simulink model "Ejemplo52"  (R2021a)
settings: Solver=ode4  StartTime=0.0  StopTime=20  FixedStep=0.01  RelTol=1e-3
settings Model: PauseTimes=10  Creator=benja  LastModifiedBy=benja

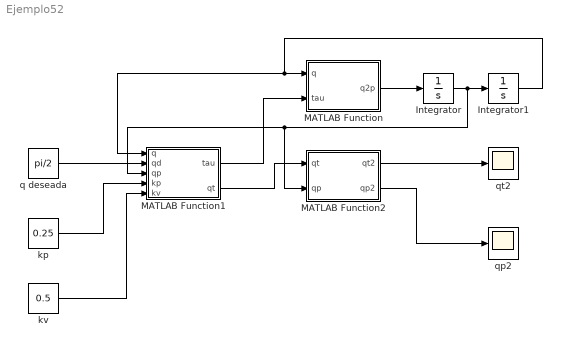
== system Ejemplo52 ==
  Integrator : Integrator
  Integrator1 : Integrator
  MATLAB Function : MATLAB Function  TreatAsAtomicUnit=on
  MATLAB Function1 : MATLAB Function  TreatAsAtomicUnit=on
  MATLAB Function2 : MATLAB Function  TreatAsAtomicUnit=on
  kp : Constant  Value=0.25
  kv : Constant  Value=0.5
  q deseada : Constant  Value=pi/2
  qp2 : Scope
  qt2 : Scope
  wires:
  MATLAB Function/1(q2p) -> Integrator/1
  Integrator/1 -> MATLAB Function2/2(qp), MATLAB Function1/3(qp), Integrator1/1
  Integrator1/1 -> MATLAB Function1/1(q), MATLAB Function/1(q)
  MATLAB Function1/1(tau) -> MATLAB Function/2(tau)
  q deseada/1 -> MATLAB Function1/2(qd)
  kp/1 -> MATLAB Function1/4(kp)
  kv/1 -> MATLAB Function1/5(kv)
  MATLAB Function2/2(qp2) -> qp2/1
  MATLAB Function1/2(qt) -> MATLAB Function2/1(qt)
  MATLAB Function2/1(qt2) -> qt2/1

== matlab function Ejemplo52/MATLAB Function1 ==
  data: q input; tau output; qd input; qp input; kp input; kv input; qt output
function [tau,qt] = fcn(q,qd,qp,kp,kv)

qt = qd - q;
tau = kp*qt-kv*qp;

== matlab function Ejemplo52/MATLAB Function ==
  data: q input; q2p output; tau input
function q2p = fcn(q,tau)

m = 1;
g = 1;
l = 1;
q2p =inv(m*l)*(tau-m*g*l*sin(q));

== matlab function Ejemplo52/MATLAB Function2 ==
  data: qt input; qt2 output; qp input; qp2 output
function [qt2,qp2] = fcn(qt,qp)

qt2 = qt^2;
qp2 = qp^2;
